simulink model "example_House_Ideal"  (R2013b)
settings: Solver=ode113  StartTime=0.0  StopTime=365*24*3600  RelTol=1e-3
libraries: carnot x7
settings Model: Creator=drhf  LastModifiedBy=drhf
settings OptimizationCC: ExpressionDepthLimit=2147483647
settings DebuggingCC: StateNameClashWarn=warning
settings GRTTargetCC: CombineOutputUpdateFcns=off  GRTInterface=on

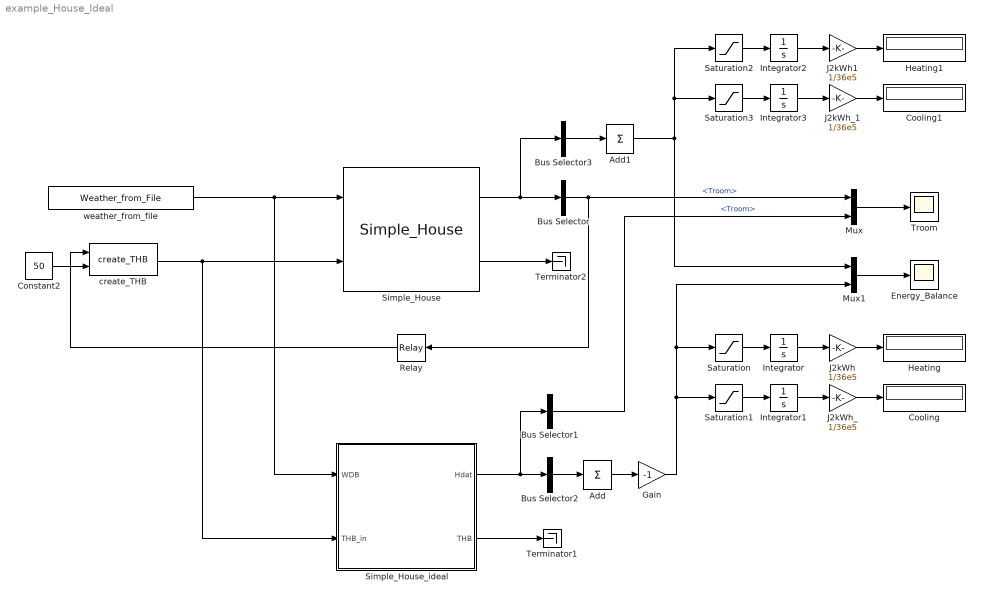
== system example_House_Ideal ==
  Add : Sum  Inputs=1
  Add1 : Sum  Inputs=1
  Bus Selector : BusSelector  OutputSignals=Troom
  Bus Selector1 : BusSelector  OutputSignals=Troom
  Bus Selector2 : BusSelector  OutputSignals=Qdot.Qdot_trans_wall,Qdot.Qdot_vent,Qdot.Qdot_ground,Qdot.Qdot_neighbour,Qdot.Qdot_internal,Qdot.Qdot_trans_window1,Qdot.Qdot_trans_window2,Qdot.Qdot_trans_window3,Qdot.Qdot_trans_window4,Qdot.Qdot_solar1,Qdot.Qdot_solar2,Qdot.Qdot_solar3,Qdot.Qdot_solar4  OutputAsBus=on
  Bus Selector3 : BusSelector  OutputSignals=Qdot.Qdot_h  OutputAsBus=on
  Constant2 : Constant  Value=50
  Cooling : Display
  Cooling1 : Display
  Energy_Balance : Scope
      settings: YMin=-3000  YMax=3000  Decimation=5
  Gain : Gain  Gain=-1
  Heating : Display
  Heating1 : Display
  Integrator{,1..3} (4 alike) : Integrator
  J2kWh : Gain  Gain=1/36e5
  J2kWh1 : Gain  Gain=1/36e5
  J2kWh_ : Gain  Gain=1/36e5
  J2kWh_1 : Gain  Gain=1/36e5
  Mux : Mux  Inputs=2
  Mux1 : Mux  Inputs=2
  Relay : Relay  OnSwitchValue=20.1  OffSwitchValue=19.9  OnOutputValue=0  OffOutputValue=800/3600
  Saturation : Saturate  UpperLimit=inf  LowerLimit=0
  Saturation1 : Saturate  UpperLimit=0  LowerLimit=-inf
  Saturation2 : Saturate  UpperLimit=inf  LowerLimit=0
  Saturation3 : Saturate  UpperLimit=0  LowerLimit=-inf
  Simple_House : carnot/Load/Houses/Simple_House  Ahabit=140  Hroom=2.6  Floorsize=[7 10]  UAwall=0.162*(54.6+26.4)+0.182*((45.7+56.0)*2 -(12+4+3+4))  UAneighbour=0  Uground=0.18  mc=0.5e6*140 % 0.5 MJ/m2/K  shade=0.75  tini=20  Awin=[12 4 3 4]  AziWin=[0 90 -180 -90]  Uwin="[1    1   1    1]*1.0"  Gwin="[1    1   1    1]*0.585*(1-0.15)"  vent=0.4  rec=0.6  heatload=1792  dpcoeff=[10 100]  delta_t_nom=15  n_rad=1.1  mass_times_cap=40e6
  Simple_House_ideal : Subsystem  mask(simple house){Ahabit=140, Hroom=2.6, Floorsize=[7 10], UAwall=0.162*(54.6+26.4)+0.182*((45.7+56.0)*2 -(12+4+3+4)), UAneighbour=0, Uground=0.18, mc=0.5e6*140 % 0.5 MJ/m2/K, Awin=[12 4 3 4], AziWin=[0 90 -180 -90], Uwin=[1    1   1    1]*1.0, Gwin=[1    1   1    1]*0.585*(1-0.15), shade=0.75, tini=20, vent=0.4, rec=0.6, uaheating=425 %400, dpcoeff=[10 100], heatload=1792, delta_t_nom=15, n_rad=1.1, mass_times_cap=40e6}
      mask prompts: Ahabit "Living surface in m²"; Hroom "height of rooms in m"; Floorsize "Dimensions of slab in m [length width]"; UAwall "Total heat transfer to ambient (walls/roof) in W/K"; UAneighbour "Total heat transfer to neighbour inW/K"; Uground "Heat transfer coeffient to ground in W/m²/K"; mc "Total thermal capacity in J/K"; Awin "Surface of 4 windows in m² (vector)"; AziWin "Orientation of 4 windows (south 0, east -90,west 90)"; Uwin "Heat loss coefficient 4 windows in W/m²/K [vector]"; Gwin "Light transmittance 4 windows (0..1) * (1 - frame_part) [vector]"; shade "Shading factor [0..1] when T room > 4 K + T_init"; tini "Initial temperature"; vent "Ventilation rate in 1/h"; rec "Heat recovery (0..1)"; uaheating "Heat transfer of the heating system in W/K"; dpcoeff "Pressure drop coefficients [linear quadratic] in Pa/(kg/s), Pa/(kg/s)²"; heatload "Heatload  [W]"; delta_t_nom "Nominal temperature difference between desired temperature and incoming THB [K]"; n_rad "Radiator exponent"; mass_times_cap "Mass*capacity of heating system [J/K]"
      mask help:
      | Simple model of 1-node room or house. The differential equation
      | (m*c)house * dT/dt = solar_gain + internal_gain + heating_power - losses_to_ambient - losses_to_neighbour_room
      | is solved.
      | The heating power is generated by a radiator or floor heating system.
      | The windows have an automatic shading (shading factor) if room temperature rises 4 K above initial temperature.
      | solar gain = Solar_Radiation_on_window * light_transmittance * shading_factor
      | Use "look under mask" to set up the models parameters (initial conditions, surfaces characteristics...).
      | A usual value for the internal gains is 2.3 W/m².
      mask init:
      | invmc = 1/mc;
      | rec = max(0,min(1,rec));
      | Gwin = max(0,min(1,Gwin));
      | shade = max(0, min(1, shade));
      mask Help: web(fullfile(path_carnot('help'),'simple_house.html'),'-helpbrowser')
      mask Display: plot(0,-15,80,100,[30,30,60,60,30],[20,50,50,20,20],[47,47,56,56,47],[40,30,30,40,40],[42,42,34,34],[20,40,40,20],[62,45,28],[48,70,48])
  Terminator1 : Terminator
  Terminator2 : Terminator
  Troom : Scope
      settings: YMin=16.5  YMax=20.75  SampleInput=on  SampleTime=3600
  create_THB : carnot/Source/Simple/create_THB  p=1e5  fluid=Water  mix=0  dia=0.02  mID=No Pressure Drop
  weather_from_file : carnot/Weather/Weather_from_File  file=DE_TRY2010_13_averageYear  ext=.mat
  wires:
  weather_from_file/1 -> Simple_House/1, Simple_House_ideal/1(WDB)
  create_THB/1 -> Simple_House/2, Simple_House_ideal/2(THB_in)
  Simple_House/1 -> Bus Selector/1, Bus Selector3/1
  Simple_House/2 -> Terminator2/1
  Bus Selector/1 -> Relay/1, Mux/1  "<Troom>"
  Simple_House_ideal/2(THB) -> Terminator1/1
  Bus Selector2/1 -> Add/1
  Simple_House_ideal/1(Hdat) -> Bus Selector1/1, Bus Selector2/1
  Add/1 -> Gain/1
  Saturation/1 -> Integrator/1
  Integrator/1 -> J2kWh/1
  Saturation1/1 -> Integrator1/1
  Integrator1/1 -> J2kWh_/1
  J2kWh/1 -> Heating/1
  J2kWh_/1 -> Cooling/1
  Bus Selector1/1 -> Mux/2  "<Troom>"
  Bus Selector3/1 -> Add1/1
  Add1/1 -> Saturation2/1, Saturation3/1, Mux1/1
  Saturation2/1 -> Integrator2/1
  Integrator2/1 -> J2kWh1/1
  Saturation3/1 -> Integrator3/1
  Integrator3/1 -> J2kWh_1/1
  J2kWh1/1 -> Heating1/1
  J2kWh_1/1 -> Cooling1/1
  Constant2/1 -> create_THB/2
  Relay/1 -> create_THB/1
  Mux/1 -> Troom/1
  Mux1/1 -> Energy_Balance/1
  Gain/1 -> Saturation1/1, Saturation/1, Mux1/2

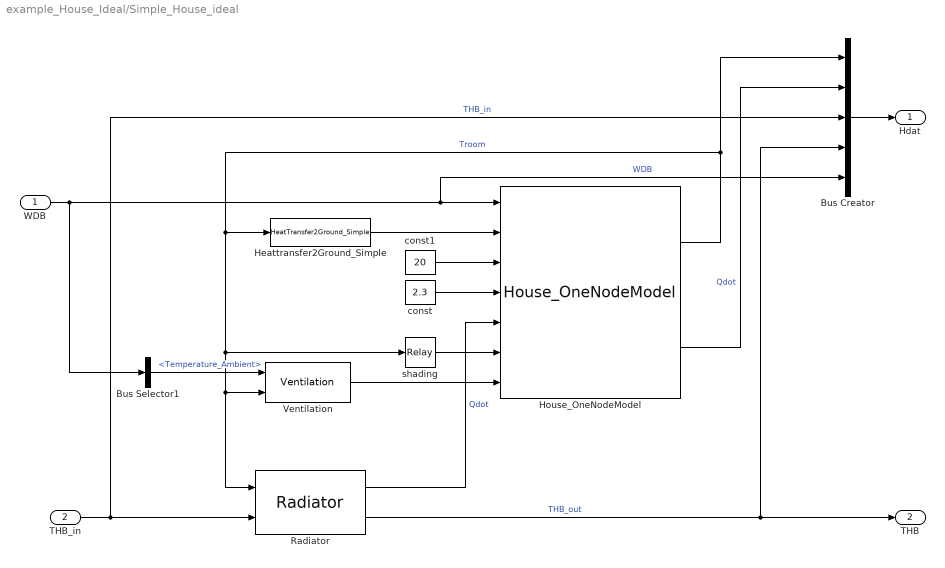
== system example_House_Ideal/Simple_House_ideal ==
  WDB : Inport
  THB_in : Inport  Port=2
  Bus Creator : BusCreator  Inputs=5
  Bus Selector1 : BusSelector  OutputSignals=Temperature_Ambient
  Heattransfer2Ground_Simple : carnot/Load/Houses/heat_transfer/HeatTransfer2Ground_Simple  Tground=10  UAground=Uground*Floorsize(1)*Floorsize(2)
  House_OneNodeModel : carnot/Basic/Thermal_Models/House_OneNodeModel  Ahabit=Ahabit  Hroom=Hroom  tini=tini  UAout=UAwall  mc=mc  UAin=UAneighbour  dtroom=0  AziWin=AziWin  Awin=Awin  Uwin=Uwin  Gwin=Gwin
  Radiator : carnot/Source/Heat_Exchanger/Radiator  pnom=heatload*1.3  dtnom=delta_t_nom  expo=n_rad  mcap=mass_times_cap  tini=tini  lin=0  qua=1000
  Ventilation : carnot/Source/Ventilation/Ventilation  vent=vent  rec=rec  Vhouse=Ahabit*Hroom
  const : Constant  Value=2.3
  const1 : Constant  Value=20
  shading : Relay  OnSwitchValue=24  OffSwitchValue=23  OnOutputValue=0.2  OffOutputValue=1
  Hdat : Outport
  THB : Outport  Port=2
  wires:
  Ventilation/1 -> House_OneNodeModel/7
  const/1 -> House_OneNodeModel/4
  shading/1 -> House_OneNodeModel/6
  House_OneNodeModel/2 -> Bus Creator/2  "Qdot"
  const1/1 -> House_OneNodeModel/3
  Bus Creator/1 -> Hdat/1
  WDB/1 -> Bus Selector1/1, Bus Creator/5, House_OneNodeModel/1  "WDB"
  THB_in/1 -> Bus Creator/3, Radiator/2  "THB_in"
  House_OneNodeModel/1 -> Bus Creator/1, shading/1, Radiator/1, Ventilation/2, Heattransfer2Ground_Simple/1  "Troom"
  Radiator/2 -> Bus Creator/4, THB/1  "THB_out"
  Radiator/1 -> House_OneNodeModel/5  "Qdot"
  Heattransfer2Ground_Simple/1 -> House_OneNodeModel/2
  Bus Selector1/1 -> Ventilation/1  "<Temperature_Ambient>"
